simulink model "untitled"  (R2021a)
settings: Solver=VariableStepAuto  StartTime=0.0  StopTime=100  RelTol=1e-3
libraries: fuzblock x1, simulink x1
settings Model: Creator=Shiva  LastModifiedBy=Shiva

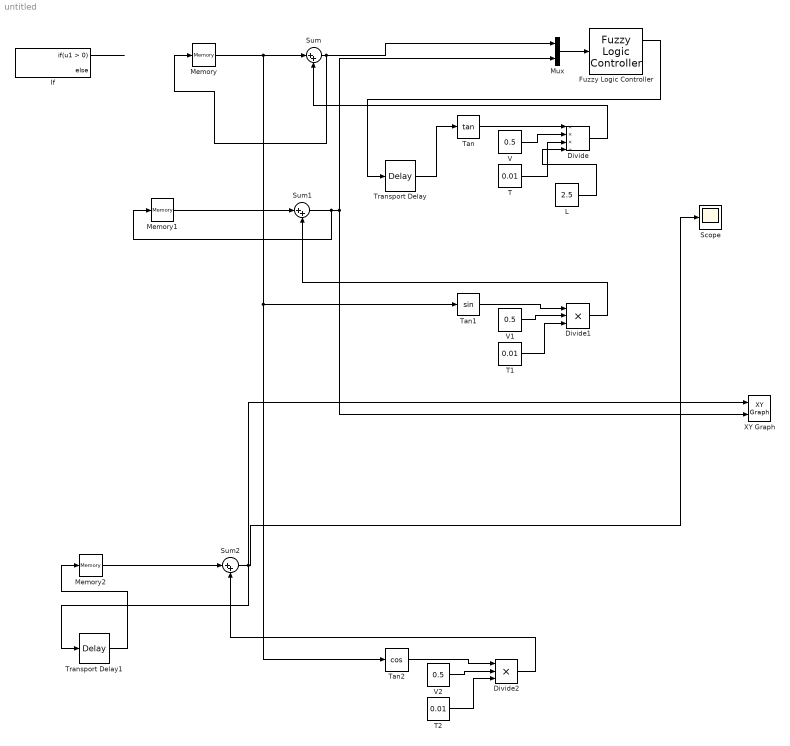
== system untitled ==
  Divide : Product  Inputs=***/
  Divide1 : Product  Inputs=***
  Divide2 : Product  Inputs=***
  Fuzzy Logic Controller : fuzblock/Fuzzy Logic  Controller  FIS=fiss_fuzzy  OutputSampleNumber=101  DataType=double  FuzzifiedInputs=off  RuleFiringStrengths=off  RuleOutputs=off  AggregatedOutputs=on  SimulateUsing=Interpreted execution  OutOfRangeInputValueMessage=warning  NoRuleFiredMessage=warning  EmptyOutputFuzzySetMessage=warning
  If : If
  L : Constant  Value=2.5
  Memory : Memory  InheritSampleTime=on  LinearizeMemory=on  LinearizeAsDelay=on
  Memory1 : Memory  InitialCondition=40  InheritSampleTime=on  LinearizeMemory=on  LinearizeAsDelay=on
  Memory2 : Memory  InitialCondition=20  LinearizeAsDelay=on
  Mux : Mux  Inputs=2
  Scope : Scope
  Sum : Sum  Inputs=|++
  Sum1 : Sum  Inputs=|++
  Sum2 : Sum  Inputs=|++
  T : Constant  Value=0.01
  T1 : Constant  Value=0.01
  T2 : Constant  Value=0.01
  Tan : Trigonometry  Operator=tan
  Tan1 : Trigonometry
  Tan2 : Trigonometry  Operator=cos
  Transport Delay : TransportDelay
  Transport Delay1 : TransportDelay
  V : Constant  Value=0.5
  V1 : Constant  Value=0.5
  V2 : Constant  Value=0.5
  XY Graph : simulink/Sinks/XY Graph  xmin=0  xmax=50  ymin=0  ymax=30  st=-1
  wires:
  Tan/1 -> Divide/1
  V/1 -> Divide/2
  T/1 -> Divide/3
  L/1 -> Divide/4
  Divide/1 -> Sum/2
  V1/1 -> Divide1/2
  Tan1/1 -> Divide1/1
  Divide1/1 -> Sum1/2
  T1/1 -> Divide1/3
  Mux/1 -> Fuzzy Logic Controller/1
  Fuzzy Logic Controller/1 -> Transport Delay/1
  Transport Delay/1 -> Tan/1
  Memory1/1 -> Sum1/1
  Sum1/1 -> Memory1/1, Mux/2, XY Graph/2
  Sum/1 -> Mux/1, Memory/1
  Divide2/1 -> Sum2/2
  Memory/1 -> Tan2/1, Tan1/1, Sum/1
  V2/1 -> Divide2/2
  Tan2/1 -> Divide2/1
  T2/1 -> Divide2/3
  Memory2/1 -> Sum2/1
  Sum2/1 -> Transport Delay1/1, XY Graph/1, Scope/1
  Transport Delay1/1 -> Memory2/1
  If/1 -> ?
